simulink model "communication_project2"  (R2021a)
settings: Solver=ode45  StartTime=0.0  StopTime=60  RelTol=1e-3  EnableMultiTasking=on
PreLoadFcn:
  | %%%%%%%%%%%%%%%%%%%%%%%%%%%%%%%%%%%%%%%%%%%%%%%%%%%%%%%%%%%%%%%%%%%%%%%%%%%
  | % check to see if Simulink library folder is missing from the MATLAB path %
  | %%%%%%%%%%%%%%%%%%%%%%%%%%%%%%%%%%%%%%%%%%%%%%%%%%%%%%%%%%%%%%%%%%%%%%%%%%%
  | if isempty(strfind(path, 'rtlsdr_book_library'))
  | 
  |     % create error window
  |     fig_error = figure(...
  |         'Name', 'Error: RTL-SDR Book Library',...
  |         'Toolbar','none',...
  |         'MenuBar','none',...
  |         'NumberTitle','off',...
  |         'Resize','off',...
  |         'WindowStyle','modal');
  |     fig_error.Position(3) = 600;
  |     fig_error.Position(4) = 150;
  |     fig_axes = axes(...
  |         'Parent',fig_error,...
  |         'Position',[0,0,1,1],...
  |         'visible','off');
  |     % error message
  |     t_title = text(.05,.8,...
  |         'MISSING DIRECTORIES',...
  |         'FontSize',11.5);
  |     t_body = text(.075,.6,...
  |         [{'Simulink cannot find the  \it{<root>}\rm / \it{rtlsdr\_book\_library}\rm  folder in the \it{MATLAB Path}\rm.'},...
  |         {'Please set the MATLAB path following the instructions given in Exercise 2.4.'}],...
  |         'FontSize',10.5);
  |     % buttons
  |     btn_path = uicontrol(...
  |         'Parent',fig_error,...
  |         'String','Set Path Now',...
  |         'FontSize',10,...
  |         'Callback', 'pathtool; close(fig_error);',...
  |         'Position', [fig_error.Position(3)/2-210, 30, 200, 30]);
  |     btn_abort = uicontrol(...
  |         'Parent',fig_error,...
  |         'String','No thanks',...
  |         'FontSize',10,...
  |         'Callback', 'close(fig_error); abort=1;',...
  |         'Position', [fig_error.Position(3)/2+10, 30, 200, 30]);
  | 
  |     % pause to allow user to interact with error box
  |     uiwait(fig_error);
  | 
  |     % abort simulation
  |     try
  |         if abort==1
  |             set_param(gcs, 'SimulationCommand', 'stop');
  |         end
  |     end
  | 
  |     % if user has set path, allow diagram to be updated
  |     if ~exist('abort','var')
  |         % create error window
  |         fig_update = figure(...
  |             'Name', 'Update Diagram',...
  |             'Toolbar','none',...
  |             'MenuBar','none',...
  |             'NumberTitle','off',...
  |             'Resize','off');
  | ... (+24 lines)
undefined symbols (not defined in the file): dfilt, fdesignblkfcn, gcbh, startfcn_spectrum_analyzer
libraries: dsparch4 x7, dspsrcs4 x2, dspvision x2, dspmlti4 x1, dspobslib x1
(part 2 of 2)

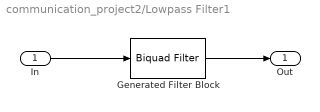
== system communication_project2/Lowpass Filter1 ==
  In : Inport
  Generated Filter Block : dsparch4/Biquad Filter  Tag=BlockMethodSubSystem  FilterSource=Dialog parameters  CoeffSource=Specify via dialog  FilterObject=BQF  IIRFiltStruct=Direct form II  BiQuadCoeffs=[0.0250565845315173404 0.0501131690630346807 0.0250565845315173404 1 -1.66183580525046892 0.923275186604771592;0.037716014607021689 0.0754320292140433779 0.037716014607021689 1 -1.56661971807023814 0.813079740544001672;0.0484945426006950717 0.0969890852013901433 0.0484945426006950717 1 -1.48383378736612204 0.717269958482403047;0.0575626893627941005 0.115125378725588201 0.0575626893627941005 1 -1.41240957564111014 0.634609316739389473;0.0650666699608493243 0.130133339921698649 0.0650666699608493243 1 -1.35133558864931036 0.563927193176257502;0.0711260498823475112 0.142252099764695022 0.0711260498823475112 1 -1.29969518746752888 0.504162743580548245;0.0758269652636444913 0.151653930527288983 0.0758269652636444913 1 -1.25668484808297043 0.454386033845194215;0.0792077080977627163 0.158415416195525433 0.0792077080977627163 1 -1.22162058776832216 0.413805477338500316;0.0812136446614236951 0.16242728932284739 0.0812136446614236951 1 -1.19393777217884889 0.381767611653830552;0.0814810648334097498 0.1629621296668195 0.0814810648334097498 1 -1.17318767708145222 0.357753119431178823;0.0766373086618705734 0.153274617323741147 0.0766373086618705734 1 -1.15903293117486372 0.341371554243555309;0.0475464966622892865 0.095092993324578573 0.0475464966622892865 1 -1.15124314512471893 0.332356281993511304;0.0454005843132187503 0.0908011686264375006 0.0454005843132187503 1 -1.14969150165554135 0.330560534559680597;0.0458312470003414685 0.091662494000682937 0.0458312470003414685 1 -1.15435274058810755 0.335955077840982497;0.0465162571239447972 0.0930325142478895944 0.0465162571239447972 1 -1.16530274620299967 0.348627734204365547;0.0474667600149336621 0.0949335200298673243 0.0474667600149336621 1 -1.18271977564157993 0.36878480413735909;0.048698191344618065 0.0973963826892361301 0.048698191344618065 1 -1.20688720946975048 0.396754249529485126;0.0502304575935993425 0.100460915187198685 0.0502304575935993425 1 -1.23819751421076951 0.432990279589241744;0.0520881013934042514 0.104176202786808503 0.0520881013934042514 1 -1.27715683093716725 0.478078661311564734;0.0543003859894366434 0.108600771978873287 0.0543003859894366434 1 -1.32438917923795718 0.532741584811574187;0.0569011931409248439 0.113802386281849688 0.0569011931409248439 1 -1.3806386047689676 0.597840148726714093;0.059928568932260555 0.11985713786452111 0.059928568932260555 1 -1.44676658326257312 0.674371355826272501;0.0634236653328399957 0.126847330665679991 0.0634236653328399957 1 -1.52374047235194654 0.763454748080988788;0.0239938368016244831 0.0479876736032489662 0.0239938368016244831 1 -1.61260659973026299 0.866301261061622974;0.0141997105327178481 0.0283994210654356961 0.0141997105327178481 1 -1.71443854044993027 0.984153364242433715;0.0284538033452553032 0.0569076066905106065 0.0284538033452553032 1 -1.63680758827266115 0.89430953998294882;0.0408317176138579402 0.0816634352277158804 0.0408317176138579402 1 -1.54480010490503439 0.787827474074976664;0.0514593923545490078 0.102918784709098016 0.0514593923545490078 1 -1.4649534370622368 0.695419358598140747;0.0605319902961252224 0.121063980592250445 0.0605319902961252224 1 -1.39620836714874419 0.615859340244761189;0.0681537712524473704 0.136307542504894741 0.0681537712524473704 1 -1.33757449136203355 0.548001205260089774;0.0744558484197530845 0.148911696839506169 0.0744558484197530845 1 -1.28816231050571739 0.490815518770047532;0.0795524795965481674 0.159104959193096335 0.0795524795965481674 1 -1.24719791450712236 0.443406619461565565;0.0835101976875831931 0.167020395375166386 0.0835101976875831931 1 -1.2140273488611264 0.405017672953716268;0.0863953604892238741 0.172790720978447748 0.0863953604892238741 1 -1.18811535156680126 0.37502921002970635;0.0882581405062864699 0.17651628101257294 0.0882581405062864699 1 -1.16904147397635549 0.352954637219240419;0.0726533405680115235 0.145306681136023047 0.0726533405680115235 1 -1.15649547260953423 0.338434903654900587;0.106312788256249069 0.212625576512498138 0.106312788256249069 1 ...(+1417 chars)]  ScaleValues=[0.0385311233339147366;1;1;1;1;1;1;1;1;1;1;1;1;1;1;1;1;1;1;1;1;1;1;1;1;1;1;1;1;1;1;1;1;1;1;1;1;1;1;1;1;1;1;1;1;1;1;1;1;1;1]  IC=0  ICnum=0  ICden=0  a0Flag=Warning  optimizeScaleValues=off  ScaleValueMode=Specify via input port (g)  InputProcessing=Columns as channels (frame based)  roundingMode=Floor  overflowMode=off  scaleValueFracLength=14  denProdOutputFracLength=30  denAccumFracLength=30  secondMemoryFracLength=15
  Out : Outport
  wires:
  In/1 -> Generated Filter Block/1
  Generated Filter Block/1 -> Out/1

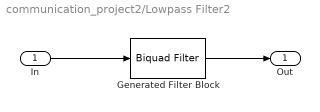
== system communication_project2/Lowpass Filter2 ==
  In : Inport
  Generated Filter Block : dsparch4/Biquad Filter  Tag=BlockMethodSubSystem  FilterSource=Dialog parameters  CoeffSource=Specify via dialog  FilterObject=BQF  IIRFiltStruct=Direct form II  BiQuadCoeffs=[0.0250565845315173404 0.0501131690630346807 0.0250565845315173404 1 -1.66183580525046892 0.923275186604771592;0.037716014607021689 0.0754320292140433779 0.037716014607021689 1 -1.56661971807023814 0.813079740544001672;0.0484945426006950717 0.0969890852013901433 0.0484945426006950717 1 -1.48383378736612204 0.717269958482403047;0.0575626893627941005 0.115125378725588201 0.0575626893627941005 1 -1.41240957564111014 0.634609316739389473;0.0650666699608493243 0.130133339921698649 0.0650666699608493243 1 -1.35133558864931036 0.563927193176257502;0.0711260498823475112 0.142252099764695022 0.0711260498823475112 1 -1.29969518746752888 0.504162743580548245;0.0758269652636444913 0.151653930527288983 0.0758269652636444913 1 -1.25668484808297043 0.454386033845194215;0.0792077080977627163 0.158415416195525433 0.0792077080977627163 1 -1.22162058776832216 0.413805477338500316;0.0812136446614236951 0.16242728932284739 0.0812136446614236951 1 -1.19393777217884889 0.381767611653830552;0.0814810648334097498 0.1629621296668195 0.0814810648334097498 1 -1.17318767708145222 0.357753119431178823;0.0766373086618705734 0.153274617323741147 0.0766373086618705734 1 -1.15903293117486372 0.341371554243555309;0.0475464966622892865 0.095092993324578573 0.0475464966622892865 1 -1.15124314512471893 0.332356281993511304;0.0454005843132187503 0.0908011686264375006 0.0454005843132187503 1 -1.14969150165554135 0.330560534559680597;0.0458312470003414685 0.091662494000682937 0.0458312470003414685 1 -1.15435274058810755 0.335955077840982497;0.0465162571239447972 0.0930325142478895944 0.0465162571239447972 1 -1.16530274620299967 0.348627734204365547;0.0474667600149336621 0.0949335200298673243 0.0474667600149336621 1 -1.18271977564157993 0.36878480413735909;0.048698191344618065 0.0973963826892361301 0.048698191344618065 1 -1.20688720946975048 0.396754249529485126;0.0502304575935993425 0.100460915187198685 0.0502304575935993425 1 -1.23819751421076951 0.432990279589241744;0.0520881013934042514 0.104176202786808503 0.0520881013934042514 1 -1.27715683093716725 0.478078661311564734;0.0543003859894366434 0.108600771978873287 0.0543003859894366434 1 -1.32438917923795718 0.532741584811574187;0.0569011931409248439 0.113802386281849688 0.0569011931409248439 1 -1.3806386047689676 0.597840148726714093;0.059928568932260555 0.11985713786452111 0.059928568932260555 1 -1.44676658326257312 0.674371355826272501;0.0634236653328399957 0.126847330665679991 0.0634236653328399957 1 -1.52374047235194654 0.763454748080988788;0.0239938368016244831 0.0479876736032489662 0.0239938368016244831 1 -1.61260659973026299 0.866301261061622974;0.0141997105327178481 0.0283994210654356961 0.0141997105327178481 1 -1.71443854044993027 0.984153364242433715;0.0284538033452553032 0.0569076066905106065 0.0284538033452553032 1 -1.63680758827266115 0.89430953998294882;0.0408317176138579402 0.0816634352277158804 0.0408317176138579402 1 -1.54480010490503439 0.787827474074976664;0.0514593923545490078 0.102918784709098016 0.0514593923545490078 1 -1.4649534370622368 0.695419358598140747;0.0605319902961252224 0.121063980592250445 0.0605319902961252224 1 -1.39620836714874419 0.615859340244761189;0.0681537712524473704 0.136307542504894741 0.0681537712524473704 1 -1.33757449136203355 0.548001205260089774;0.0744558484197530845 0.148911696839506169 0.0744558484197530845 1 -1.28816231050571739 0.490815518770047532;0.0795524795965481674 0.159104959193096335 0.0795524795965481674 1 -1.24719791450712236 0.443406619461565565;0.0835101976875831931 0.167020395375166386 0.0835101976875831931 1 -1.2140273488611264 0.405017672953716268;0.0863953604892238741 0.172790720978447748 0.0863953604892238741 1 -1.18811535156680126 0.37502921002970635;0.0882581405062864699 0.17651628101257294 0.0882581405062864699 1 -1.16904147397635549 0.352954637219240419;0.0726533405680115235 0.145306681136023047 0.0726533405680115235 1 -1.15649547260953423 0.338434903654900587;0.106312788256249069 0.212625576512498138 0.106312788256249069 1 ...(+1417 chars)]  ScaleValues=[0.0385311233339147366;1;1;1;1;1;1;1;1;1;1;1;1;1;1;1;1;1;1;1;1;1;1;1;1;1;1;1;1;1;1;1;1;1;1;1;1;1;1;1;1;1;1;1;1;1;1;1;1;1;1]  IC=0  ICnum=0  ICden=0  a0Flag=Warning  optimizeScaleValues=off  ScaleValueMode=Specify via input port (g)  InputProcessing=Columns as channels (frame based)  roundingMode=Floor  overflowMode=off  scaleValueFracLength=14  denProdOutputFracLength=30  denAccumFracLength=30  secondMemoryFracLength=15
  Out : Outport
  wires:
  Generated Filter Block/1 -> Out/1
  In/1 -> Generated Filter Block/1
